simulink model "DT_UDE"  (R2019b)
settings: Solver=ode4  StartTime=0.0  StopTime=tstop  FixedStep=tstep  RelTol=1e-3
values from neighbouring files (symbols this model uses):
  b = 0.7    [data.m]
  tstep = 0.01    [data.m]
  xhat_ic = [-1 -2]    [data.m]
  xic = [-2 1]    [data.m]
settings Model: Creator=Ram Padmanabhan  LastModifiedBy=Maithili Shetty
settings DataIOCC: SaveOutput=off  SignalLogging=off  DSMLogging=off  SaveTime=off  ReturnWorkspaceOutputs=off

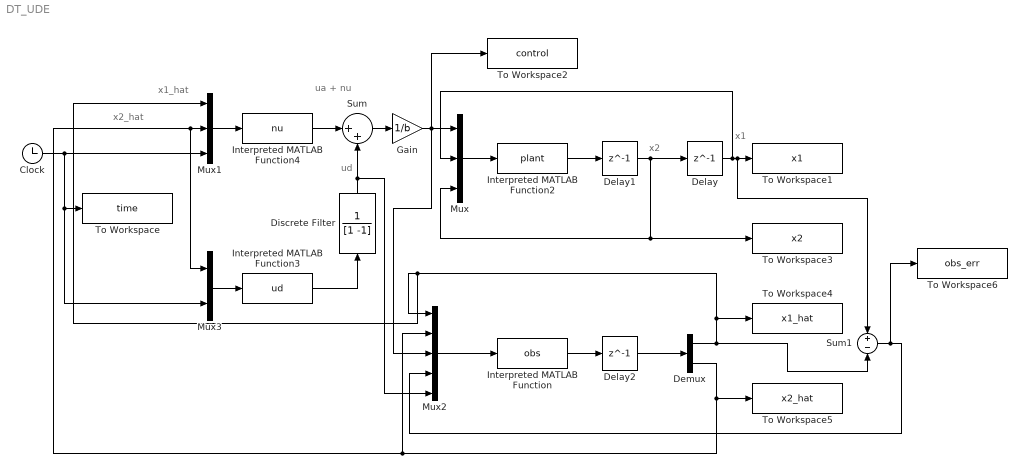
== system DT_UDE ==
  note: ud
  note: x2_hat
  note: x1_hat
  note: x1
  note: x2
  note: ua + nu
  Clock : Clock
  Delay : Delay  DelayLength=1  InitialCondition=xic(1)  SampleTime=tstep
  Delay1 : Delay  DelayLength=1  InitialCondition=xic(2)  SampleTime=tstep
  Delay2 : Delay  DelayLength=1  InitialCondition=xhat_ic  SampleTime=tstep
  Demux : Demux  Outputs=2
  Discrete Filter : DiscreteFilter  Numerator=1  Denominator=[1 -1]  SampleTime=tstep
  Gain : Gain  Gain=1/b
  Interpreted MATLAB Function : MATLABFcn  MATLABFcn=obs  OutputDimensions=2
  Interpreted MATLAB Function2 : MATLABFcn  MATLABFcn=plant  OutputDimensions=1
  Interpreted MATLAB Function3 : MATLABFcn  MATLABFcn=ud  OutputDimensions=1
  Interpreted MATLAB Function4 : MATLABFcn  MATLABFcn=nu  OutputDimensions=1
  Mux : Mux  Inputs=3
  Mux1 : Mux  Inputs=3
  Mux2 : Mux  Inputs=5
  Mux3 : Mux  Inputs=2
  Sum : Sum  Inputs=|++
  Sum1 : Sum  Inputs=+-
  To Workspace : ToWorkspace  VariableName=time  SampleTime=-1
  To Workspace1 : ToWorkspace  VariableName=x1  SampleTime=-1
  To Workspace2 : ToWorkspace  VariableName=control  SampleTime=-1
  To Workspace3 : ToWorkspace  VariableName=x2  SampleTime=-1
  To Workspace4 : ToWorkspace  VariableName=x1_hat  SampleTime=-1
  To Workspace5 : ToWorkspace  VariableName=x2_hat  SampleTime=-1
  To Workspace6 : ToWorkspace  VariableName=obs_err  SampleTime=-1
  wires:
  Delay1/1 -> Delay/1, Mux/3, To Workspace3/1
  Interpreted MATLAB Function2/1 -> Delay1/1
  Mux/1 -> Interpreted MATLAB Function2/1
  Delay/1 -> Sum1/1, To Workspace1/1, Mux/2
  Mux1/1 -> Interpreted MATLAB Function4/1
  Clock/1 -> Mux1/3, Mux3/2, To Workspace/1
  Mux3/1 -> Interpreted MATLAB Function3/1
  Interpreted MATLAB Function3/1 -> Discrete Filter/1
  Interpreted MATLAB Function4/1 -> Sum/1
  Discrete Filter/1 -> Mux2/5, Sum/2
  Mux2/1 -> Interpreted MATLAB Function/1
  Interpreted MATLAB Function/1 -> Delay2/1
  Delay2/1 -> Demux/1
  Demux/1 -> Sum1/2, To Workspace4/1, Mux1/1, Mux2/1
  Demux/2 -> To Workspace5/1, Mux3/1, Mux1/2, Mux2/2
  Sum/1 -> Gain/1
  Gain/1 -> Mux2/3, To Workspace2/1, Mux/1
  Sum1/1 -> To Workspace6/1, Mux2/4
